simulink model "SCARAHybCtrl"  (R2023b)
settings: Solver=ode15s  StartTime=0.0  StopTime=20  RelTol=1e-3
values from neighbouring files (symbols this model uses):
  dq0 = [0.0; 0.0; 0.0]    [init.m]
  env_damping = 150.0    (= 150)    [init.m]
  env_stiffness = 15000.0    (= 15000)    [init.m]
  g = 9.807    [init.m]
  Kad_f = 25.0    (= 25)    [init.m]
  Kd_p = diag([25.0, 25.0, 0.0])    [init.m]
  Ki_f = diag([0.0, 0.0, 0.0])    [init.m]
  Kp_f = diag([0.0, 0.0, 2.0])    [init.m]
  Kp_p = diag([50.0, 50.0, 0.0])    [init.m]
  L1 = 0.300    (= 0.3)    [init.m]
  L2 = 0.250    (= 0.25)    [init.m]
  m_load = 1.1    [init.m]
  N = 50    [init.m]
  q0 = [1.1251; 1.6081; 0.0]    [init.m]
  z_surface = 0.0    (= 0)    [init.m]
undefined symbols (not defined in the file or in its folder): fric_params_ctrl, Im2_eq, Im3_eq, pi_1, pi_2, pi_3, pi_4, pi_5
libraries: simulink x1
settings Model: Creator=davi_  LastModifiedBy=davi_

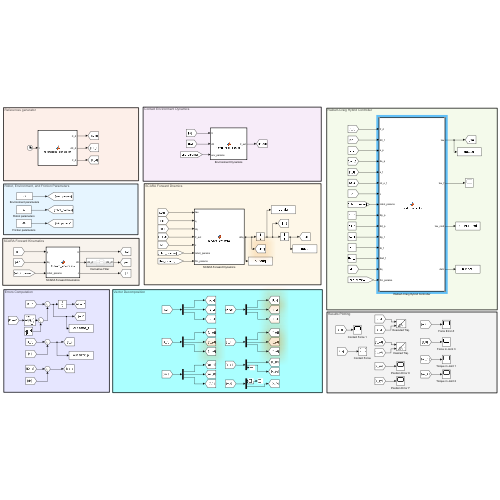
[thumbnail: Simulink's stored preview of the top-level diagram]
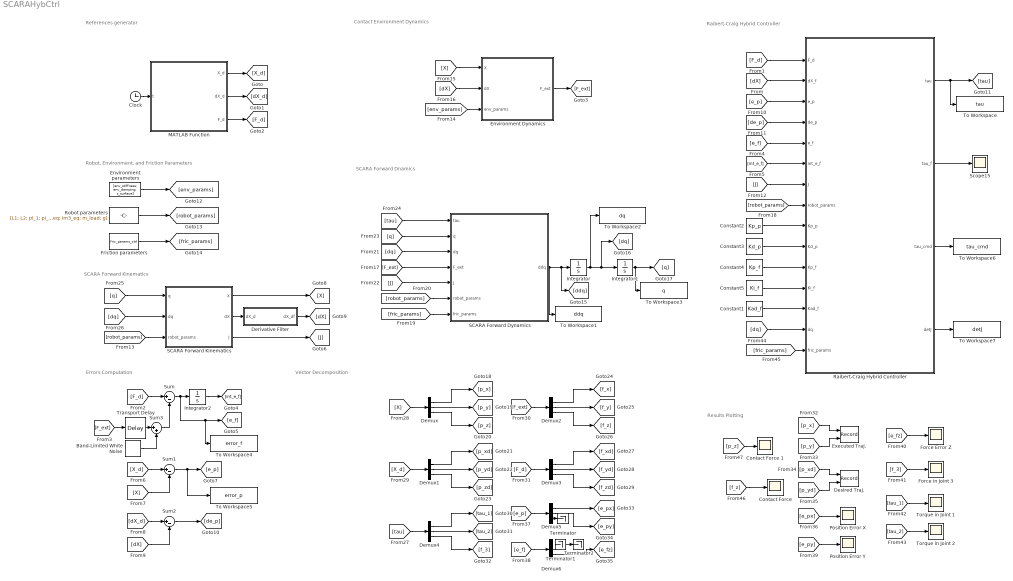
== system SCARAHybCtrl ==
  note: Results Plotting
  note: Vector Decomposition
  note: Robot, Environment, and Friction Parameters
  note: SCARA Forward Dnamics
  note: SCARA Forward Kinematics
  note: Contact Environment Dynamics
  note: Raibert-Craig Hybrid Controller
  note: References generator
  note: Errors Computation
  Band-Limited White Noise : simulink/Sources/Band-Limited White Noise  Cov=[0.0025]  Ts=0.01  seed=[23341]
  Clock : Clock
  Constant1 : Constant  Value=Kad_f  VectorParams1D=off
  Constant2 : Constant  Value=Kp_p  VectorParams1D=off
  Constant3 : Constant  Value=Kd_p  VectorParams1D=off
  Constant4 : Constant  Value=Kp_f  VectorParams1D=off
  Constant5 : Constant  Value=Ki_f  VectorParams1D=off
  "Contact Force " : Scope
  Contact Force 1 : Scope
  Demux{,1..6} (7 alike) : Demux  Outputs=3
  Derivative Filter : Subsystem
  Desired Traj. : Record  FileSettingsInternal="{\"entries\":[{\"content\":{\"excelSettings\":{\"content\":{},\"type\":\"Streamout.ExcelSettings\"}},\"type\":\"Streamout.FileSettingStorage\",\"uuid\":\"\"}],\"packageUris\":[\"http:\\/\\/schema.mathworks.com\\/mf0\\/streamout_blocks\\/R2020a\"],\"version\":\"1.0\"}"  Layout=[1 1]  SignalsInternal="{\"entries\":[{\"content\":{\"signals\":[{\"content\":{\"blockPath\":[],\"dimensions\":[1,1],\"domain\":\"\",\"lineColor\":\"#a2142f\",\"plots\":[1],\"port\":1,\"sid\":[\"\"],\"signalID\":771,\"signalName\":\"From34\"},\"type\":\"RecordBlkView.Signal\",\"uuid\":\"\"},{\"content\":{\"blockPath\":[],\"dimensions\":[1,1],\"domain\":\"\",\"lineColor\":\"#139fff\",\"plots\":[1],\"port\":2,\"sid\":[\"\"],\"signalID\":775,\"signalName\":\"From35\"},\"type\":\"RecordBlkView.Signal\",\"uuid\":\"\"}]},\"type\":\"RecordBlkView.InputSignals\",\"uuid\":\"\"}],\"packageUris\":[\"http:\\/\\/schema.mathworks.com\\/mf0\\/streamout_blocks\\/R2020a\"],\"version\":\"1.0\"}"  VisualizationBindings="{\"xyplotplugin\":{\"info\":[{\"series\":[{\"bindingParametersList\":[{\"parameter\":\"X-Axis\",\"signalID\":771,\"signalName\":\"From34\"},{\"parameter\":\"Y-Axis\",\"signalID\":775,\"signalName\":\"From35\"}],\"seriesID\":35207}],\"subplotID\":1}]}}"  CompatibilityTag=XY
  Environment Dynamics : MATLAB Function  TreatAsAtomicUnit=on
  Environment parameters : Constant  Value=[env_stiffness; env_damping; z_surface]  VectorParams1D=off
  Executed Traj. : Record  FileSettingsInternal="{\"entries\":[{\"content\":{\"excelSettings\":{\"content\":{},\"type\":\"Streamout.ExcelSettings\"}},\"type\":\"Streamout.FileSettingStorage\",\"uuid\":\"\"}],\"packageUris\":[\"http:\\/\\/schema.mathworks.com\\/mf0\\/streamout_blocks\\/R2020a\"],\"version\":\"1.0\"}"  Layout=[1 1]  SignalsInternal="{\"entries\":[{\"content\":{\"signals\":[{\"content\":{\"blockPath\":[],\"dimensions\":[1,1],\"domain\":\"\",\"lineColor\":\"#ff6929\",\"plots\":[1],\"port\":1,\"sid\":[\"\"],\"signalID\":779,\"signalName\":\"From32\"},\"type\":\"RecordBlkView.Signal\",\"uuid\":\"\"},{\"content\":{\"blockPath\":[],\"dimensions\":[1,1],\"domain\":\"\",\"lineColor\":\"#b746ff\",\"plots\":[1],\"port\":2,\"sid\":[\"\"],\"signalID\":783,\"signalName\":\"From33\"},\"type\":\"RecordBlkView.Signal\",\"uuid\":\"\"}]},\"type\":\"RecordBlkView.InputSignals\",\"uuid\":\"\"}],\"packageUris\":[\"http:\\/\\/schema.mathworks.com\\/mf0\\/streamout_blocks\\/R2020a\"],\"version\":\"1.0\"}"  VisualizationBindings="{\"xyplotplugin\":{\"info\":[{\"series\":[{\"bindingParametersList\":[{\"parameter\":\"X-Axis\",\"signalID\":779,\"signalName\":\"From32\"},{\"parameter\":\"Y-Axis\",\"signalID\":783,\"signalName\":\"From33\"}],\"seriesID\":48668}],\"subplotID\":1}]}}"  CompatibilityTag=XY
  Force Error Z : Scope
  Force in Joint 3 : Scope
  Friction parameters : Constant  Value=fric_params_ctrl  VectorParams1D=off
  Integrator : Integrator  InitialCondition=dq0
  Integrator1 : Integrator  InitialCondition=q0
  Integrator2 : Integrator  InitialCondition=q0
  MATLAB Function : MATLAB Function  TreatAsAtomicUnit=on
  Position Error X : Scope
  Position Error Y : Scope
  Raibert-Craig Hybrid Controller : MATLAB Function  TreatAsAtomicUnit=on
  Robot parameters : Constant  Value=[L1; L2; pi_1; pi_2; pi_3; pi_4; pi_5; Im2_eq; Im3_eq; m_load; g]  VectorParams1D=off
  SCARA Forward Dynamics : MATLAB Function  TreatAsAtomicUnit=on
  SCARA Forward Kinematics : MATLAB Function  TreatAsAtomicUnit=on
  Scope15 : Scope
  Sum : Sum  Inputs=|+-
  Sum1 : Sum  Inputs=|+-
  Sum2 : Sum  Inputs=|+-
  Sum3 : Sum  Inputs=|++
  Terminator : Terminator
  Terminator1 : Terminator
  Terminator2 : Terminator
  To Workspace : ToWorkspace  VariableName=tau  SampleTime=-1
  To Workspace1 : ToWorkspace  VariableName=ddq  SampleTime=-1
  To Workspace2 : ToWorkspace  VariableName=dq  SampleTime=-1
  To Workspace3 : ToWorkspace  VariableName=q  SampleTime=-1
  To Workspace4 : ToWorkspace  VariableName=error_f  SampleTime=-1
  To Workspace5 : ToWorkspace  VariableName=error_p  SampleTime=-1
  To Workspace6 : ToWorkspace  VariableName=tau_cmd  SampleTime=-1
  To Workspace7 : ToWorkspace  VariableName=detJ  SampleTime=-1
  Torque in Joint 1 : Scope
  Torque in Joint 2 : Scope
  Transport Delay : TransportDelay  DelayTime=0.005
  wires:
  SCARA Forward Dynamics/1(ddq) -> [ddq], Integrator/1, To Workspace1/1
  Integrator/1 -> To Workspace2/1, [dq], Integrator1/1
  Environment Dynamics/1(F_ext) -> [F_ext]
  Raibert-Craig Hybrid Controller/1(tau) -> To Workspace/1, [tau]
  Constant2/1 -> Raibert-Craig Hybrid Controller/9(Kp_p)
  Constant3/1 -> Raibert-Craig Hybrid Controller/10(Kd_p)
  Constant4/1 -> Raibert-Craig Hybrid Controller/11(Kp_f)
  Constant5/1 -> Raibert-Craig Hybrid Controller/12(Ki_f)
  Clock/1 -> MATLAB Function/1(t)
  Raibert-Craig Hybrid Controller/2(tau_f) -> Scope15/1
  Constant1/1 -> Raibert-Craig Hybrid Controller/13(Kad_f)
  MATLAB Function/1(X_d) -> [X_d]
  MATLAB Function/2(dX_d) -> [dX_d]
  MATLAB Function/3(F_d) -> [F_d]
  [F_d] -> Raibert-Craig Hybrid Controller/1(F_d)
  Integrator2/1 -> [int_e_f]
  Sum/1 -> To Workspace4/1, [e_f], Integrator2/1
  [F_d] -> Sum/1
  [e_f] -> Raibert-Craig Hybrid Controller/5(e_f)
  [int_e_f] -> Raibert-Craig Hybrid Controller/6(int_e_f)
  [X] -> Sum1/2
  [X_d] -> Sum1/1
  Sum1/1 -> To Workspace5/1, [e_p]
  SCARA Forward Kinematics/1(X) -> [X]
  SCARA Forward Kinematics/2(dX) -> Derivative Filter/1(dX_d)
  Derivative Filter/1(dX_df) -> [dX]
  [dX_d] -> Sum2/1
  Sum2/1 -> [de_p]
  [dX] -> Sum2/2
  [dX] -> Raibert-Craig Hybrid Controller/2(dX_f)
  [e_p] -> Raibert-Craig Hybrid Controller/3(e_p)
  [de_p] -> Raibert-Craig Hybrid Controller/4(de_p)
  SCARA Forward Kinematics/3(J) -> [J]
  [J] -> Raibert-Craig Hybrid Controller/7(J)
  Environment parameters/1 -> [env_params]
  Robot parameters/1 -> [robot_params]
  Friction parameters/1 -> [fric_params]
  [robot_params] -> SCARA Forward Kinematics/3(robot_params)
  [env_params] -> Environment Dynamics/3(env_params)
  [X] -> Environment Dynamics/1(X)
  [dX] -> Environment Dynamics/2(dX)
  Integrator1/1 -> To Workspace3/1, [q]
  [robot_params] -> Raibert-Craig Hybrid Controller/8(robot_params)
  [fric_params] -> SCARA Forward Dynamics/7(fric_params)
  [robot_params] -> SCARA Forward Dynamics/6(robot_params)
  [J] -> SCARA Forward Dynamics/5(J)
  [F_ext] -> SCARA Forward Dynamics/4(F_ext)
  [dq] -> SCARA Forward Dynamics/3(dq)
  [q] -> SCARA Forward Dynamics/2(q)
  [tau] -> SCARA Forward Dynamics/1(tau)
  [q] -> SCARA Forward Kinematics/1(q)
  [dq] -> SCARA Forward Kinematics/2(dq)
  [X] -> Demux/1
  [X_d] -> Demux1/1
  Demux/1 -> [p_x]
  Demux/2 -> [p_y]
  Demux/3 -> [p_z]
  Demux1/1 -> [p_xd]
  Demux1/2 -> [p_yd]
  Demux1/3 -> [p_zd]
  Demux2/1 -> [f_x]
  Demux2/2 -> [f_y]
  Demux2/3 -> [f_z]
  Demux3/3 -> [f_zd]
  Demux3/2 -> [f_yd]
  Demux3/1 -> [f_xd]
  [F_d] -> Demux3/1
  [F_ext] -> Demux2/1
  Demux4/3 -> [f_3]
  Demux4/2 -> [tau_2]
  Demux4/1 -> [tau_1]
  [tau] -> Demux4/1
  [p_x] -> Executed Traj./1
  [p_y] -> Executed Traj./2
  [p_xd] -> Desired Traj./1
  [p_yd] -> Desired Traj./2
  [e_px] -> Position Error X/1
  [e_p] -> Demux5/1
  Demux5/1 -> [e_px]
  Demux5/2 -> [e_py]
  Demux5/3 -> Terminator/1
  [e_f] -> Demux6/1
  Demux6/2 -> Terminator2/1
  Demux6/3 -> [e_fz]
  [e_py] -> Position Error Y/1
  [e_fz] -> Force Error Z/1
  [f_3] -> Force in Joint 3/1
  [tau_2] -> Torque in Joint 2/1
  [tau_1] -> Torque in Joint 1/1
  Raibert-Craig Hybrid Controller/3(tau_cmd) -> To Workspace6/1
  [dq] -> Raibert-Craig Hybrid Controller/14(dq)
  [fric_params] -> Raibert-Craig Hybrid Controller/15(fric_params)
  [f_z] -> "Contact Force "/1
  [F_ext] -> Transport Delay/1
  Transport Delay/1 -> Sum3/1
  Band-Limited White Noise/1 -> Sum3/2
  Sum3/1 -> Sum/2
  [p_z] -> Contact Force 1/1
  Raibert-Craig Hybrid Controller/4(detJ) -> To Workspace7/1

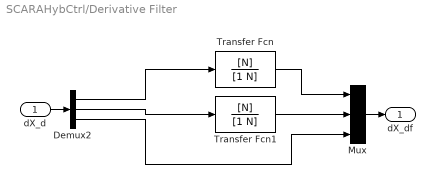
== system SCARAHybCtrl/Derivative Filter ==
  dX_d : Inport
  Demux2 : Demux  Outputs=3
  Mux : Mux  Inputs=3
  Transfer Fcn : TransferFcn  Numerator=[N]  Denominator=[1 N]
  Transfer Fcn1 : TransferFcn  Numerator=[N]  Denominator=[1 N]
  dX_df : Outport
  wires:
  Transfer Fcn1/1 -> Mux/2
  Transfer Fcn/1 -> Mux/1
  Demux2/3 -> Mux/3
  dX_d/1 -> Demux2/1
  Demux2/2 -> Transfer Fcn1/1
  Mux/1 -> dX_df/1
  Demux2/1 -> Transfer Fcn/1

== matlab function SCARAHybCtrl/Environment Dynamics ==
  data: X input; F_ext output; dX input; env_params input
function F_ext = kelvin_voigt_contact(X, dX, env_params)
    % """
    % Computes the external contact force using a unilateral Kelvin-Voigt model.
    %
    % This function simulates a rigid ground surface. It evaluates the current
    % Cartesian position and velocity of the end-effector. If penetration into
    % the surface occurs, it applies a viscoelastic restoring force. The contact
    % is strictly unilateral (the ground can push, but cannot pull).
    %
    % Args:
    %     X (3x1 column vector): Cartesian position of the end-effector [x; y; z].
    %     dX (3x1 column vector): Cartesian velocity of the end-effector [dx; dy; dz].
    %     env_params (3x1 column vector): Environment parameters 
    %                                     [stiffness; damping; z_surface].
    %
    % Returns:
    %     F_ext (3x1 column vector): External force vector applied to the 
    %                                end-effector [Fx; Fy; Fz].
    % """

    % Extract Z-axis states
    z = X(3);
    dz = dX(3);
    
    % Extract environment parameters
    Ke = env_params(1);
    Be = env_params(2);
    z_sup = env_params(3);
    
    % Initialize Z-axis force
    Fz = 0.0;
    
    % Check for penetration (contact condition)
    if z <= z_sup
        % Viscoelastic force: Stiffness * penetration_depth - Damping * velocity
        Fz = Ke * (z_sup - z) - Be * dz;
        
        % Unilateral constraint: The ground cannot pull the end-effector
        if Fz < 0.0
            Fz = 0.0;
        end
    end
    
    % Assemble the 3x1 external force vector (acting only on the Z-axis)
    F_ext = [0.0; 0.0; Fz];

end

== matlab function SCARAHybCtrl/SCARA Forward Kinematics ==
  data: q input; X output; dq input; robot_params input; dX output; J output
function [X, dX, J] = forward_kinematics(q, dq, robot_params)
    % """
    % Computes the forward kinematics and analytical Jacobian for a 3-DOF SCARA.
    %
    % This geometric model is matched to the DH parameters of the Omron Adept 550
    % (Boschetti & Sinico, 2025, Table 1). It calculates the end-effector's 
    % Cartesian position, velocity, and the 3x3 analytical Jacobian matrix.
    %
    % Args:
    %     q (3x1 column vector): Current joint positions [q1 (rad); q2 (rad); d3 (m)].
    %     dq (3x1 column vector): Current joint velocities [dq1; dq2; dd3].
    %     L (2x1 column vector): Link lengths [L1; L2] in meters.
    %
    % Returns:
    %     X (3x1 column vector): Cartesian position of the end-effector [x; y; z].
    %     dX (3x1 column vector): Cartesian velocity of the end-effector [dx; dy; dz].
    %     J (3x3 matrix): Analytical Jacobian matrix (dX = J * dq).
    % """
    
    % Extract individual joint variables
    q1 = q(1);
    q2 = q(2);
    q3 = q(3);
    
    % Extract link lengths
    L1 = robot_params(1);
    L2 = robot_params(2);
    
    % Precompute trigonometric terms to optimize simulation speed
    c1 = cos(q1);
    s1 = sin(q1);
    c12 = cos(q1 + q2);
    s12 = sin(q1 + q2);
    
    % 1. Forward Kinematics (Position X)
    % Planar 2R kinematics for X and Y; direct mapping for prismatic Z
    x = L1 * c1 + L2 * c12;
    y = L1 * s1 + L2 * s12;
    z = q3; 
    
    X = [x; y; z];
    
    % 2. Analytical Jacobian Matrix (J)
    % Row 1: Partial derivatives of x with respect to q1, q2, q3
    J11 = -L1 * s1 - L2 * s12;
    J12 = -L2 * s12;
    J13 = 0.0;
    
    % Row 2: Partial derivatives of y with respect to q1, q2, q3
    J21 = L1 * c1 + L2 * c12;
    J22 = L2 * c12;
    J23 = 0.0;
    
    % Row 3: Partial derivatives of z with respect to q1, q2, q3
    J31 = 0.0;
    J32 = 0.0;
    J33 = 1.0;
    
    J = [J11, J12, J13;
         J21, J22, J23;
         J31, J32, J33];
         
    % 3. Cartesian Velocity (dX)
    dX = J * dq;
end

== matlab function SCARAHybCtrl/SCARA Forward Dynamics ==
  data: tau input; ddq output; q input; dq input; F_ext input; J input; robot_params input; fric_params input
function ddq = forward_dynamics(tau, q, dq, F_ext, J, robot_params, fric_params)
    % """
    % Computes the forward dynamics of the Omron 550 SCARA robot.
    %
    % This function calculates the joint accelerations (ddq) given the applied
    % joint torques, current states, external contact forces, and the analytical
    % Jacobian. The dynamic model uses LUMPED PARAMETERS derived from
    % Boschetti and Sinico (2025), specifically Table 7.
    % """
    
    % 1. Parameter Extraction (Lumped Parameters)
    a1     = robot_params(1); % L1
    a2     = robot_params(2); % L2
    pi_1   = robot_params(3); % m2*a1^2 + Im1_eq + J1_zz
    pi_2   = robot_params(4); % m2*c2x
    pi_3   = robot_params(5); % J2_zz + J3_zz
    pi_4   = robot_params(6); % m3 (Z-axis link mass)
    pi_5   = robot_params(7); % J4_zz
    Im2_eq = robot_params(8);
    Im3_eq = robot_params(9);
    M_load = robot_params(10);
    g0     = robot_params(11);
    
    B_visc = fric_params(1:3);
    F_coulomb = fric_params(4:6);
    
    % Total moving mass on Z-axis
    m3_tot = pi_4 + M_load;
    
    % 2. States and Trigonometry
    dq1 = dq(1); 
    dq2 = dq(2); 
    c2  = cos(q(2));
    s2  = sin(q(2));
    
    % 3. Inertia Matrix M(q) (Using Lumped Equations A11 - A13)
    % Eq. A11: m11
    m11 = pi_1 + pi_3 + pi_5 + (a1^2 + a2^2)*m3_tot + 2*a1*c2*(pi_2 + a2*m3_tot);
          
    % Eq. A12: m12 and m21
    m12 = pi_3 + pi_5 + a2*m3_tot*(a2 + a1*c2) + a1*pi_2*c2;
    
    % Eq. A13/A5 equivalent: m22 
    % Note: The theoretical c2x^2*m2 term is naturally absorbed by J2_zz (pi_3)
    % via the Huygens-Steiner (parallel axis) theorem.
    m22 = pi_3 + pi_5 + (a2^2)*m3_tot + Im2_eq;
    
    % Eq. A6: m33
    m33 = m3_tot + Im3_eq;
    
    M_matrix = [m11, m12, 0.0;
                m12, m22, 0.0;
                0.0, 0.0, m33];
                
    % 4. Coriolis Matrix C(q, dq) (Equations A8 and A9)
    c11 = -a1 * s2 * (a2*m3_tot + pi_2) * (2*dq1*dq2 + dq2^2);
    c21 = (dq1^2) * a1 * s2 * (a2*m3_tot + pi_2);
    
    C_vector = [c11; c21; 0.0];
    
    % 5. Gravity Vector g(q) (Z-up operational space)
    g31 = g0 * m3_tot; 
    
    G_vector = [0.0; 0.0; g31];
    
    % 6. Friction Torque Vector
    v_th = 0.05; 
    tau_fric = B_visc .* dq + F_coulomb .* tanh(dq / v_th);
    
    % 7. Calculation of Accelerations (ddq)
    rhs = tau - C_vector - G_vector - tau_fric + (J' * F_ext);
    ddq = M_matrix \ rhs;
end

== matlab function SCARAHybCtrl/Raibert-Craig Hybrid Controller ==
  data: F_d input; dX_f input; e_p input; tau output; de_p input; e_f input; int_e_f input; J input; robot_params input; Kp_p input; Kd_p input; Kp_f input; Ki_f input; tau_f output; Kad_f input; tau_cmd output; dq input; fric_params input; detJ output
function [tau, tau_f, tau_cmd, detJ] = hybrid_controller(F_d, dX_f, e_p, de_p, e_f, int_e_f, J, robot_params, Kp_p, Kd_p, Kp_f, Ki_f, Kad_f, dq, fric_params)
    % """
    % Implements the Raibert-Craig Hybrid Position/Force Controller
    % with Gravity and Friction Feedforward Compensation.
    % """
    detJ = 0.0;
    
    % 1. Selection Matrices
    S = diag([1.0, 1.0, 0.0]);
    I_S = diag([0.0, 0.0, 1.0]); 
    
    % 2. Position Control Loop (PD)
    tau_p = Kp_p * e_p + Kd_p * de_p;
    
    % 3. Force Control Loop (PI + Active Damping)
    tau_f = -F_d - Kp_f * e_f - Ki_f * int_e_f - [0; 0; Kad_f * dX_f(3)];
    
    % 4. Gravity Compensation (Static - Z Axis Only)
    pi_4   = robot_params(6);  
    M_load = robot_params(10); 
    g      = robot_params(11); 
    m3_tot = pi_4 + M_load;
    G_vector = [0.0; 0.0; m3_tot * g];
    
    % 5. Friction Feedforward Compensation
    B_visc = fric_params(1:3);
    F_coulomb = fric_params(4:6);
    v_th = 0.05;
    
    % Friction compensation
    tau_fric_comp = B_visc .* dq + F_coulomb .* tanh(dq / v_th);
    
    % 6. Operational to Joint Space Mapping
    tau_cmd = (J') * (S * tau_p + I_S * tau_f) + G_vector + tau_fric_comp;
    tau = tau_cmd;
    
    % 7. Actuator Saturation Protection
    tau1_max = 60.0;  
    tau2_max = 30.0;  
    tau3_max = 150.0; 
    
    tau(1) = min(max(tau(1), -tau1_max), tau1_max);
    tau(2) = min(max(tau(2), -tau2_max), tau2_max);
    tau(3) = min(max(tau(3), -tau3_max), tau3_max);

    detJ = J(1,1)*J(2,2) - J(1,2)*J(2,1);
end

== matlab function SCARAHybCtrl/MATLAB Function ==
  data: t input; X_d output; dX_d output; F_d output
function [X_d, dX_d, F_d] = references_generator(t)
    % """
    % Generates a high-density trochoidal reference trajectory and force step for polishing.
    % """
    
    % 1. Time Parameterization (Quintic Smoothing)
    T_total = 20.0; 
    t_c = min(t, T_total);  
    tau = t_c / T_total;    
    
    s = 10*tau^3 - 15*tau^4 + 6*tau^5;
    ds_dtau = 30*tau^2 - 60*tau^3 + 30*tau^4;
    ds_dt = ds_dtau / T_total;
    
    % 2. Trochoidal Path Geometry 
    x_start = -0.100;
    x_end   =  0.100;
    L_pass  = x_end - x_start;
    y_center = 0.350;  
    
    R = 0.040;
    num_loops = 5;
    
    % 3. Position Equations
    x_feed = x_start + L_pass * s;
    dx_feed = L_pass * ds_dt;
    
    theta = 2 * pi * num_loops * s;
    dtheta = 2 * pi * num_loops * ds_dt;
    
    x_d = x_feed + R * sin(theta);
    y_d = y_center + R * cos(theta);
    z_d = 0.0;
    
    % 4. Velocity Equations (Chain Rule)
    dx_d = dx_feed + R * cos(theta) * dtheta;
    dy_d = -R * sin(theta) * dtheta;
    dz_d = 0.0;
    
    % 5. Force Dynamics (Z-Axis)
    target_force = 25.0;  
    ramp_duration = 1.5;
    if t < ramp_duration
        Fz_d = (target_force / ramp_duration) * t;
    else
        Fz_d = target_force;
    end
    
    % 6. Output Assembly
    X_d = [x_d; y_d; z_d];
    dX_d = [dx_d; dy_d; dz_d];
    F_d = [0.0; 0.0; Fz_d];
end
